simulink model "estimation_velocity"  (R2023b)
settings: Solver=FixedStepDiscrete  StartTime=0.0  StopTime=10.0  FixedStep=EstimationVelocity_Ts  RelTol=1e-3  EnableMultiTasking=on
model workspace (MAT data in the model file):
  EstimationVelocity_Ts = Simulink.Parameter
  EstimationVelocity_Ts.Value = 0.001
  EstimationVelocity_Ts.DataType = 'auto'
  EstimationVelocity_Ts.DocUnits = 's'
  EstimationVelocity_Ts.Complexity = 'real'
  EstimationVelocity_Ts.Dimensions = [1 1]
libraries: dspbuff3 x1, dsppolyfun x1
settings Model: DataDictionary=newBoard.sldd  Creator=ascalzo  LastModifiedBy=mfussi
settings SolverCC: AllowMultiTaskInputOutput=on  AutoInsertRateTranBlk=on  InsertRTBMode=Never (minimum delay)
settings DataIOCC: SaveOutput=off  SignalLogging=off  DSMLogging=off  SaveTime=off  ReturnWorkspaceOutputs=off
settings OptimizationCC: DefaultParameterBehavior=Inlined  DefaultUnderspecifiedDataType=single  StrengthReduction=on  PassReuseOutputArgsAs=Individual arguments  OptimizeBlockOrder=speed  OptimizationPriority=Speed  OptimizationCustomize=off  MultiThreadedLoops=on  EfficientTunableParamExpr=on
settings DebuggingCC: ParameterPrecisionLossMsg=none  UnconnectedInputMsg=warning  UnconnectedOutputMsg=warning  UnconnectedLineMsg=warning
settings HardwareCC: ProdBitPerPointer=32  ProdBitPerSizeT=32  ProdBitPerPtrDiffT=32  ProdLargestAtomicInteger=Long  ProdLargestAtomicFloat=Double  ProdWordSize=32  ProdHWDeviceType=ARM Compatible->ARM Cortex-M
settings ModelReferenceCC: UpdateModelReferenceTargets=Force  EnableRefExpFcnMdlSchedulingChecks=on
settings SFSimCC: MATLABDynamicMemAlloc=off
settings RTWCC: Description=Embedded Coder  SystemTargetFile=ert.tlc  GenCodeOnly=on  PackageGeneratedCodeAndArtifacts=on  PackageName=estimation_velocity  TemplateMakefile=ert_default_tmf  TargetLang=C++  DLArmComputeVersion=19.05
settings CodeAppCC: ForceParamTrailComments=on  IgnoreCustomStorageClasses=off  MaxIdLength=60  OperatorAnnotations=on  SimulinkDataObjDesc=on  SFDataObjDesc=on  InsertBlockDesc=on
settings ERTTargetCC: TargetLangStandard=C++03 (ISO)  CodeReplacementLibrary=ARM Cortex-M,iCubTech  GenerateSampleERTMain=on  CodeInterfacePackaging=Reusable function  InlinedParameterPlacement=NonHierarchical  RootIOFormat=Structure reference  ERTCustomFileTemplate=example_file_process.tlc

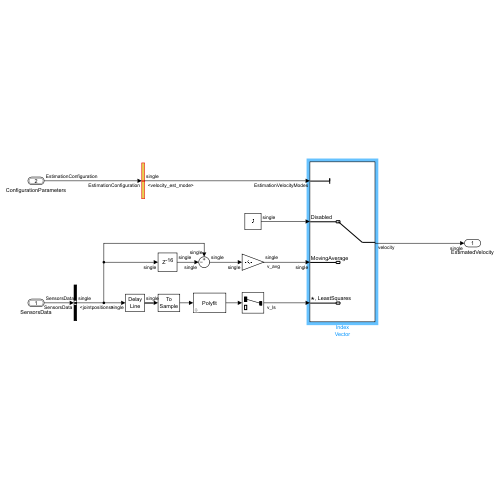
[thumbnail: Simulink's stored preview of the top-level diagram]
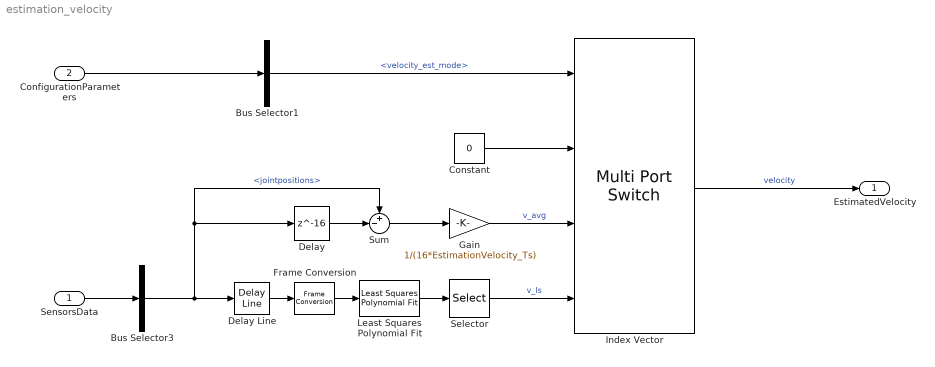
== system estimation_velocity ==
  SensorsData : Inport  OutDataTypeStr=Bus: SensorsData  BusOutputAsStruct=on
  ConfigurationParameters : Inport  Port=2  OutDataTypeStr=Bus: EstimationConfiguration  BusOutputAsStruct=on
  Bus Selector1 : BusSelector  OutputSignals=velocity_est_mode
  Bus Selector3 : BusSelector  OutputSignals=jointpositions
  Constant : Constant  Value=0  OutDataTypeStr=single
  Delay : Delay  DelayLength=16  UseCircularBuffer=on
  Delay Line : dspbuff3/Delay Line  siz=16  ic=0  directfeed=on  enable_output=off  hold_output=off  OutputFrames=on
  Frame Conversion : FrameConversion  OutFrame=Sample-based
  Gain : Gain  Gain=1/(16*EstimationVelocity_Ts)
  Index Vector : MultiPortSwitch  DataPortOrder=Specify indices  DataPortIndices={EstimationVelocityModes.Disabled, EstimationVelocityModes.MovingAverage, EstimationVelocityModes.LeastSquares}  DiagnosticForDefault=None  SaturateOnIntegerOverflow=off  InputSameDT=off
  Least Squares Polynomial Fit : dsppolyfun/Least Squares Polynomial Fit  X=(0:15) * EstimationVelocity_Ts  N=1
  Selector : Selector  InputPortWidth=2  IndexOptions=Index vector (dialog)  Indices=1  OutputSizes=1
  Sum : Sum  Inputs=+-|
  EstimatedVelocity : Outport  OutDataTypeStr=single  Unit=deg/s  LockScale=on  BusOutputAsStruct=on
  wires:
  SensorsData/1 -> Bus Selector3/1
  Bus Selector3/1 -> Sum/1, Delay/1, Delay Line/1  "<jointpositions>"
  Delay Line/1 -> Frame Conversion/1
  Sum/1 -> Gain/1
  Least Squares Polynomial Fit/1 -> Selector/1
  Delay/1 -> Sum/2
  Frame Conversion/1 -> Least Squares Polynomial Fit/1
  Gain/1 -> Index Vector/3  "v_avg"
  Selector/1 -> Index Vector/4  "v_ls"
  ConfigurationParameters/1 -> Bus Selector1/1
  Index Vector/1 -> EstimatedVelocity/1  "velocity"
  Constant/1 -> Index Vector/2
  Bus Selector1/1 -> Index Vector/1  "<velocity_est_mode>"
